simulink model "FormulaElectric"  (R2015a)
settings: Solver=ode1  StartTime=0.0  StopTime=inf  FixedStep=0.001  RelTol=1e-3
InitFcn:
  | %init_dyn_platform
  | FEParameters
StartFcn:
  | tic
StopFcn:
  | toc
undefined symbols (not defined in the file): Battery, Env, magnitude, Motor, RPM2Rad
libraries: vehicleLib x22, mblibv1 x15, driveline x12, fl_lib x8, simulink x6, AMKMotor x4, nesl_utility x4, WheelAssembly x4, ephysenetlib x2, ControllerLib x1, simulink_extras x1
(part 3 of 4)

== system FormulaElectric/Vehicle_model/Import Parameters ==
  Bus Creator1 : BusCreator  Inputs=934
  S-Function : S-Function  FunctionName=carparameters
      mask Display:
      | A=fileread('carparameters.h');
      | p=0;
      | namen=[];
      | for k=4:length(A)-5;
      |     if strcmp(A(k:k+4),'float')&~strcmp(A(k-3:k+4),'// float')&~strcmp(A(k-2:k+4),'//float')
      |         l=0;
      |         isfound=0;
      |         while ~isfound
      |             l=l+1;
      |             isfound=strcmp(A(k+l),';');
      |         end %while
      |         name=A(k+6:k+l-1);
      |         if strcmp(A(k+l-20:k+l-1),'[CAR_PARAM_MAXWHEEL]');
      |             name=A(k+6:k+l-21);
      |             for m=0:3
      |                 p=p+1;
      |                 port_label('output',p,[name,num2str(m)])
      |             end %for
      |         elseif strcmp(A(k+l-3:k+l-1),'[3]');
      |             name=A(k+6:k+l-4);
      |             p=p+1;
      |                 port_label('output',p,[name,'x'])
      |             p=p+1;
      |                 port_label('output',p,[name,'y'])
      |             p=p+1;
      |                 port_label('output',p,[name,'z'])
      |         elseif strcmp(A(k+l-3:k+l-1),'[7]');
      |             name=A(k+6:k+l-4);
      |             for m=0:6
      |                 p=p+1;
      |                 port_label('output',p,[name,num2str(m)])
      |             end
      |         elseif strcmp(A(k+l-16:k+l-1),'[INERTIA_TENSOR]');
      |             if  strcmp(A(k+l-36:k+l-1),'[CAR_PARAM_MAXWHEEL][INERTIA_TENSOR]');
      |             name=A(k+6:k+l-37);
      |             for n=0:3
      |             for m=0:5
      |                 p=p+1;
      |                 port_label('output',p,[name,num2str(n),num2str(m)])
      |             end
      |             end
      |             else
      |             name=A(k+6:k+l-17);
      |             for m=0:5
      |                 p=p+1;
      |                 port_label('output',p,[name,num2str(m)])
      |             end
      |             end %if
      |         elseif strcmp(A(k+l-20:k+l-1),'[PLANKPOINTS][THREE]');
      |             name=A(k+6:k+l-21);
      |             for m=0:7
      |             p=p+1;
      |                 port_label('output',p,[name,num2str(m),'x'])
      |             p=p+1;
      |                 port_label('output',p,[name,num2str(m),'y'])
      |             p=p+1;
      |                 port_label('output',p,[name,num2str(m),'z'])
      |             end
      |         else
      |         p=p+1;
      |         port_label('output',p,name)
      |         end %if
      |         %port_label('output',p,name)
      |     end %if
      | end %for
  imPar : Outport
  wires:
  S-Function/8 -> Bus Creator1/8  "aeroRefArea"
  S-Function/934 -> Bus Creator1/934  "test5"
  S-Function/933 -> Bus Creator1/933  "test4"
  S-Function/932 -> Bus Creator1/932  "test3"
  S-Function/931 -> Bus Creator1/931  "test2"
  S-Function/927 -> Bus Creator1/927  "suspThresholdDeg1"
  S-Function/928 -> Bus Creator1/928  "suspThresholdDeg2"
  S-Function/929 -> Bus Creator1/929  "suspThresholdDeg3"
  S-Function/930 -> Bus Creator1/930  "test1"
  S-Function/1 -> Bus Creator1/1  "bodyMass"
  S-Function/2 -> Bus Creator1/2  "bodyIxx"
  S-Function/3 -> Bus Creator1/3  "bodyIyy"
  S-Function/4 -> Bus Creator1/4  "bodyIzz"
  S-Function/5 -> Bus Creator1/5  "totVehMass"
  S-Function/6 -> Bus Creator1/6  "bodyCGz"
  S-Function/7 -> Bus Creator1/7  "aeroRho"
  S-Function/9 -> Bus Creator1/9  "aeroRefCX"
  S-Function/10 -> Bus Creator1/10  "aeroRefCZF"
  S-Function/11 -> Bus Creator1/11  "aeroRefCZR"
  S-Function/12 -> Bus Creator1/12  "aeroRefRHF"
  S-Function/13 -> Bus Creator1/13  "aeroRefRHR"
  S-Function/14 -> Bus Creator1/14  "aeroPxF"
  S-Function/15 -> Bus Creator1/15  "aeroPyF"
  S-Function/16 -> Bus Creator1/16  "aeroPzF"
  S-Function/18 -> Bus Creator1/18  "aeroPyR"
  S-Function/19 -> Bus Creator1/19  "aeroPzR"
  S-Function/20 -> Bus Creator1/20  "brakeBiasRatio"
  S-Function/21 -> Bus Creator1/21  "brakeMaxP"
  S-Function/22 -> Bus Creator1/22  "brakeDMasterF"
  S-Function/23 -> Bus Creator1/23  "brakeDiF"
  S-Function/24 -> Bus Creator1/24  "brakeDoF"
  S-Function/25 -> Bus Creator1/25  "brakeMuF"
  S-Function/26 -> Bus Creator1/26  "brakeBiasRatioF"
  S-Function/27 -> Bus Creator1/27  "brakeTCapF"
  S-Function/28 -> Bus Creator1/28  "brakeT0F"
  S-Function/29 -> Bus Creator1/29  "brakeTConF"
  S-Function/30 -> Bus Creator1/30  "brakeDCalF"
  S-Function/31 -> Bus Creator1/31  "brakeDiR"
  S-Function/32 -> Bus Creator1/32  "brakeDoR"
  S-Function/33 -> Bus Creator1/33  "brakeMuR"
  S-Function/34 -> Bus Creator1/34  "brakeBiasRatioR"
  S-Function/35 -> Bus Creator1/35  "brakeTCapR"
  S-Function/36 -> Bus Creator1/36  "brakeT0R"
  S-Function/37 -> Bus Creator1/37  "brakeTConR"
  S-Function/38 -> Bus Creator1/38  "brakeDCalR"
  S-Function/39 -> Bus Creator1/39  "steerR"
  S-Function/40 -> Bus Creator1/40  "steerPinionR"
  S-Function/41 -> Bus Creator1/41  "steerLeftMax"
  S-Function/42 -> Bus Creator1/42  "steerRightMax"
  S-Function/43 -> Bus Creator1/43  "steerDamper"
  S-Function/44 -> Bus Creator1/44  "steerStiff"
  S-Function/45 -> Bus Creator1/45  "steerPowerA"
  S-Function/46 -> Bus Creator1/46  "steerPowerTc"
  S-Function/47 -> Bus Creator1/47  "steerPMin"
  S-Function/48 -> Bus Creator1/48  "steerPMax"
  S-Function/49 -> Bus Creator1/49  "steerPowerZoneLeft"
  S-Function/50 -> Bus Creator1/50  "steerPowerZoneRight"
  S-Function/51 -> Bus Creator1/51  "engineMass"
  S-Function/52 -> Bus Creator1/52  "engineInertiaXX"
  S-Function/53 -> Bus Creator1/53  "engineInertiaYY"
  S-Function/54 -> Bus Creator1/54  "engineInertiaZZ"
  S-Function/55 -> Bus Creator1/55  "engineDamp"
  S-Function/56 -> Bus Creator1/56  "engineIdleSp"
  S-Function/57 -> Bus Creator1/57  "engineMaxTorq"
  S-Function/58 -> Bus Creator1/58  "clutchFCloseUp"
  S-Function/59 -> Bus Creator1/59  "clutchFCloseDown"
  S-Function/60 -> Bus Creator1/60  "clutchNbPlates"
  S-Function/61 -> Bus Creator1/61  "gearNbGears"
  S-Function/62 -> Bus Creator1/62  "gearEff"
  S-Function/63 -> Bus Creator1/63  "gearShiftTimeUp"
  S-Function/64 -> Bus Creator1/64  "gearShiftTimeDown"
  S-Function/65 -> Bus Creator1/65  "gearRatioPrim"
  S-Function/66 -> Bus Creator1/66  "gearRatio0"
  S-Function/67 -> Bus Creator1/67  "gearRatio1"
  S-Function/68 -> Bus Creator1/68  "gearRatio2"
  S-Function/69 -> Bus Creator1/69  "gearRatio3"
  S-Function/70 -> Bus Creator1/70  "gearRatio4"
  S-Function/71 -> Bus Creator1/71  "gearRatio5"
  S-Function/72 -> Bus Creator1/72  "gearRatio6"
  S-Function/73 -> Bus Creator1/73  "gearRatio7"
  S-Function/74 -> Bus Creator1/74  "diffType0"
  S-Function/75 -> Bus Creator1/75  "diffType1"
  S-Function/76 -> Bus Creator1/76  "diffType2"
  S-Function/77 -> Bus Creator1/77  "diffRatio0"
  S-Function/78 -> Bus Creator1/78  "diffRatio1"
  S-Function/79 -> Bus Creator1/79  "diffRatio2"
  S-Function/80 -> Bus Creator1/80  "diffPAngle0"
  S-Function/81 -> Bus Creator1/81  "diffPAngle1"
  S-Function/82 -> Bus Creator1/82  "diffPAngle2"
  S-Function/83 -> Bus Creator1/83  "diffCAngle0"
  S-Function/84 -> Bus Creator1/84  "diffCAngle1"
  S-Function/85 -> Bus Creator1/85  "diffCAngle2"
  S-Function/86 -> Bus Creator1/86  "diffClutch0"
  S-Function/87 -> Bus Creator1/87  "diffClutch1"
  S-Function/88 -> Bus Creator1/88  "diffClutch2"
  S-Function/89 -> Bus Creator1/89  "diffLock0"
  S-Function/90 -> Bus Creator1/90  "diffLock1"
  S-Function/91 -> Bus Creator1/91  "diffLock2"
  S-Function/92 -> Bus Creator1/92  "suspStiff0"
  S-Function/93 -> Bus Creator1/93  "suspStiff1"
  S-Function/94 -> Bus Creator1/94  "suspStiff2"
  S-Function/95 -> Bus Creator1/95  "suspStiff3"
  S-Function/96 -> Bus Creator1/96  "suspSpringRestLength0"
  S-Function/97 -> Bus Creator1/97  "suspSpringRestLength1"
  S-Function/98 -> Bus Creator1/98  "suspSpringRestLength2"
  S-Function/99 -> Bus Creator1/99  "suspSpringRestLength3"
  S-Function/100 -> Bus Creator1/100  "suspDamp0"
  S-Function/101 -> Bus Creator1/101  "suspDamp1"
  S-Function/102 -> Bus Creator1/102  "suspDamp2"
  S-Function/103 -> Bus Creator1/103  "suspDamp3"
  S-Function/104 -> Bus Creator1/104  "suspDampLength0"
  S-Function/105 -> Bus Creator1/105  "suspDampLength1"
  S-Function/106 -> Bus Creator1/106  "suspDampLength2"
  S-Function/107 -> Bus Creator1/107  "suspDampLength3"
  S-Function/108 -> Bus Creator1/108  "suspRimMass0"
  S-Function/109 -> Bus Creator1/109  "suspRimMass1"
  S-Function/110 -> Bus Creator1/110  "suspRimMass2"
  S-Function/111 -> Bus Creator1/111  "suspRimMass3"
  S-Function/112 -> Bus Creator1/112  "suspRimRadius0"
  S-Function/113 -> Bus Creator1/113  "suspRimRadius1"
  S-Function/114 -> Bus Creator1/114  "suspRimRadius2"
  S-Function/115 -> Bus Creator1/115  "suspRimRadius3"
  S-Function/116 -> Bus Creator1/116  "suspRimInertiaXX0"
  S-Function/117 -> Bus Creator1/117  "suspRimInertiaXX1"
  S-Function/118 -> Bus Creator1/118  "suspRimInertiaXX2"
  S-Function/119 -> Bus Creator1/119  "suspRimInertiaXX3"
  S-Function/120 -> Bus Creator1/120  "suspRimInertiaYY0"
  S-Function/121 -> Bus Creator1/121  "suspRimInertiaYY1"
  S-Function/122 -> Bus Creator1/122  "suspRimInertiaYY2"
  S-Function/123 -> Bus Creator1/123  "suspRimInertiaYY3"
  S-Function/124 -> Bus Creator1/124  "suspRimInertiaZZ0"
  S-Function/125 -> Bus Creator1/125  "suspRimInertiaZZ1"
  S-Function/126 -> Bus Creator1/126  "suspRimInertiaZZ2"
  S-Function/127 -> Bus Creator1/127  "suspRimInertiaZZ3"
  S-Function/128 -> Bus Creator1/128  "suspCamber0"
  S-Function/129 -> Bus Creator1/129  "suspCamber1"
  S-Function/130 -> Bus Creator1/130  "suspCamber2"
  S-Function/131 -> Bus Creator1/131  "suspCamber3"
  S-Function/132 -> Bus Creator1/132  "suspCaster0"
  S-Function/133 -> Bus Creator1/133  "suspCaster1"
  S-Function/134 -> Bus Creator1/134  "suspCaster2"
  S-Function/135 -> Bus Creator1/135  "suspCaster3"
  S-Function/136 -> Bus Creator1/136  "suspToe0"
  S-Function/137 -> Bus Creator1/137  "suspToe1"
  S-Function/138 -> Bus Creator1/138  "suspToe2"
  S-Function/139 -> Bus Creator1/139  "suspToe3"
  S-Function/140 -> Bus Creator1/140  "suspRH0"
  S-Function/141 -> Bus Creator1/141  "suspRH1"
  S-Function/142 -> Bus Creator1/142  "suspRH2"
  S-Function/143 -> Bus Creator1/143  "suspRH3"
  S-Function/144 -> Bus Creator1/144  "suspTr0"
  S-Function/145 -> Bus Creator1/145  "suspTr1"
  S-Function/146 -> Bus Creator1/146  "suspTr2"
  S-Function/147 -> Bus Creator1/147  "suspTr3"
  S-Function/148 -> Bus Creator1/148  "suspPrel0"
  S-Function/149 -> Bus Creator1/149  "suspPrel1"
  S-Function/150 -> Bus Creator1/150  "suspPrel2"
  S-Function/151 -> Bus Creator1/151  "suspPrel3"
  S-Function/152 -> Bus Creator1/152  "suspAttFz"
  S-Function/153 -> Bus Creator1/153  "suspAttRz"
  S-Function/154 -> Bus Creator1/154  "suspRollCF"
  S-Function/155 -> Bus Creator1/155  "suspRollCR"
  S-Function/156 -> Bus Creator1/156  "suspRollPosF"
  S-Function/157 -> Bus Creator1/157  "suspRollPosR"
  S-Function/158 -> Bus Creator1/158  "tyreMass0"
  S-Function/159 -> Bus Creator1/159  "tyreMass1"
  S-Function/160 -> Bus Creator1/160  "tyreMass2"
  S-Function/161 -> Bus Creator1/161  "tyreMass3"
  S-Function/162 -> Bus Creator1/162  "tyreRadius0"
  S-Function/163 -> Bus Creator1/163  "tyreRadius1"
  S-Function/164 -> Bus Creator1/164  "tyreRadius2"
  S-Function/165 -> Bus Creator1/165  "tyreRadius3"
  S-Function/166 -> Bus Creator1/166  "tyreInertiaXX0"
  S-Function/167 -> Bus Creator1/167  "tyreInertiaXX1"
  S-Function/168 -> Bus Creator1/168  "tyreInertiaXX2"
  S-Function/169 -> Bus Creator1/169  "tyreInertiaXX3"
  S-Function/170 -> Bus Creator1/170  "tyreInertiaYY0"
  S-Function/171 -> Bus Creator1/171  "tyreInertiaYY1"
  S-Function/172 -> Bus Creator1/172  "tyreInertiaYY2"
  S-Function/173 -> Bus Creator1/173  "tyreInertiaYY3"
  S-Function/174 -> Bus Creator1/174  "tyreInertiaZZ0"
  S-Function/175 -> Bus Creator1/175  "tyreInertiaZZ1"
  S-Function/176 -> Bus Creator1/176  "tyreInertiaZZ2"
  S-Function/177 -> Bus Creator1/177  "tyreInertiaZZ3"
  S-Function/178 -> Bus Creator1/178  "tyreLfz0f"
  S-Function/179 -> Bus Creator1/179  "tyreLcxf"
  S-Function/180 -> Bus Creator1/180  "tyreLmuxf"
  S-Function/181 -> Bus Creator1/181  "tyreLexf"
  S-Function/182 -> Bus Creator1/182  "tyreLkxf"
  S-Function/183 -> Bus Creator1/183  "tyreLhxf"
  S-Function/184 -> Bus Creator1/184  "tyreLvxf"
  S-Function/185 -> Bus Creator1/185  "tyreLcyf"
  S-Function/186 -> Bus Creator1/186  "tyreLmuyf"
  S-Function/187 -> Bus Creator1/187  "tyreLeyf"
  S-Function/188 -> Bus Creator1/188  "tyreLkyf"
  S-Function/189 -> Bus Creator1/189  "tyreLkycf"
  S-Function/190 -> Bus Creator1/190  "tyreLkzcf"
  S-Function/191 -> Bus Creator1/191  "tyreLhyf"
  S-Function/192 -> Bus Creator1/192  "tyreLvyf"
  S-Function/193 -> Bus Creator1/193  "tyreLtrf"
  S-Function/194 -> Bus Creator1/194  "tyreLresf"
  S-Function/195 -> Bus Creator1/195  "tyreLxalf"
  S-Function/196 -> Bus Creator1/196  "tyreLykaf"
  S-Function/197 -> Bus Creator1/197  "tyreLvykaf"
  S-Function/198 -> Bus Creator1/198  "tyreLsf"
  S-Function/199 -> Bus Creator1/199  "tyreLmxf"
  S-Function/200 -> Bus Creator1/200  "tyreLvmxf"
  S-Function/201 -> Bus Creator1/201  "tyreLmyf"
  S-Function/202 -> Bus Creator1/202  "tyreLmpf"
  S-Function/203 -> Bus Creator1/203  "tyreLsgkpf"
  S-Function/204 -> Bus Creator1/204  "tyreLsgalf"
  S-Function/205 -> Bus Creator1/205  "tyreLdampf"
  S-Function/206 -> Bus Creator1/206  "tyreLmassf"
  S-Function/207 -> Bus Creator1/207  "tyreLInertiaf"
  S-Function/208 -> Bus Creator1/208  "tyreEnableChkF"
  S-Function/209 -> Bus Creator1/209  "tyreEnableSatF"
  S-Function/210 -> Bus Creator1/210  "tyreEnableTempF"
  S-Function/211 -> Bus Creator1/211  "tyreTempAF"
  S-Function/212 -> Bus Creator1/212  "tyreTempBF"
  S-Function/213 -> Bus Creator1/213  "tyreLfz0r"
  S-Function/214 -> Bus Creator1/214  "tyreLcxr"
  S-Function/215 -> Bus Creator1/215  "tyreLmuxr"
  S-Function/216 -> Bus Creator1/216  "tyreLexr"
  S-Function/217 -> Bus Creator1/217  "tyreLkxr"
  S-Function/218 -> Bus Creator1/218  "tyreLhxr"
  S-Function/219 -> Bus Creator1/219  "tyreLvxr"
  S-Function/220 -> Bus Creator1/220  "tyreLcyr"
  S-Function/221 -> Bus Creator1/221  "tyreLmuyr"
  S-Function/222 -> Bus Creator1/222  "tyreLeyr"
  S-Function/223 -> Bus Creator1/223  "tyreLkyr"
  S-Function/224 -> Bus Creator1/224  "tyreLkycr"
  S-Function/225 -> Bus Creator1/225  "tyreLkzcr"
  S-Function/226 -> Bus Creator1/226  "tyreLhyr"
  S-Function/227 -> Bus Creator1/227  "tyreLvyr"
  S-Function/228 -> Bus Creator1/228  "tyreLtrr"
  S-Function/229 -> Bus Creator1/229  "tyreLresr"
  S-Function/230 -> Bus Creator1/230  "tyreLxalr"
  S-Function/231 -> Bus Creator1/231  "tyreLykar"
  S-Function/232 -> Bus Creator1/232  "tyreLvykar"
  S-Function/233 -> Bus Creator1/233  "tyreLsr"
  S-Function/234 -> Bus Creator1/234  "tyreLmxr"
  S-Function/235 -> Bus Creator1/235  "tyreLvmxr"
  S-Function/236 -> Bus Creator1/236  "tyreLmyr"
  S-Function/237 -> Bus Creator1/237  "tyreLmpr"
  S-Function/238 -> Bus Creator1/238  "tyreLsgkpr"
  S-Function/239 -> Bus Creator1/239  "tyreLsgalr"
  S-Function/240 -> Bus Creator1/240  "tyreLdampr"
  S-Function/241 -> Bus Creator1/241  "tyreLmassr"
  S-Function/242 -> Bus Creator1/242  "tyreLInertiar"
  S-Function/243 -> Bus Creator1/243  "tyreEnableChkR"
  S-Function/244 -> Bus Creator1/244  "tyreEnableSatR"
  S-Function/245 -> Bus Creator1/245  "tyreEnableTempR"
  S-Function/246 -> Bus Creator1/246  "tyreTempAR"
  S-Function/247 -> Bus Creator1/247  "tyreTempBR"
  S-Function/248 -> Bus Creator1/248  "CSantiStallMode"
  S-Function/249 -> Bus Creator1/249  "CSantiStallEnable"
  S-Function/250 -> Bus Creator1/250  "CSantiStallRPM"
  S-Function/251 -> Bus Creator1/251  "CSantiStallTime"
  S-Function/252 -> Bus Creator1/252  "CStracContrKp"
  S-Function/253 -> Bus Creator1/253  "CStracContrKi"
  S-Function/254 -> Bus Creator1/254  "CStracContrMinVel"
  S-Function/255 -> Bus Creator1/255  "CSthrPulseEnableUp"
  S-Function/256 -> Bus Creator1/256  "CSthrPulseEnableDown"
  S-Function/257 -> Bus Creator1/257  "CSthrPulseKp"
  S-Function/258 -> Bus Creator1/258  "CSthrPulseKi"
  S-Function/259 -> Bus Creator1/259  "CSidleConThrLim"
  S-Function/260 -> Bus Creator1/260  "CSidleConRPM"
  S-Function/261 -> Bus Creator1/261  "CSidleConMinRPM"
  S-Function/262 -> Bus Creator1/262  "CSidleConMaxRPM"
  S-Function/263 -> Bus Creator1/263  "CSidleConKp"
  S-Function/264 -> Bus Creator1/264  "CSidleConKi"
  S-Function/17 -> Bus Creator1/17  "aeroPxR"
  S-Function/265 -> Bus Creator1/265  "CSpitLimVel"
  S-Function/266 -> Bus Creator1/266  "skidLongF"
  S-Function/267 -> Bus Creator1/267  "skidLatF"
  S-Function/268 -> Bus Creator1/268  "skidLongR"
  S-Function/269 -> Bus Creator1/269  "skidLatR"
  S-Function/270 -> Bus Creator1/270  "clutchMaxPedalDispl"
  S-Function/271 -> Bus Creator1/271  "clutchMaxDispl"
  S-Function/272 -> Bus Creator1/272  "clutchFOpenUp"
  S-Function/273 -> Bus Creator1/273  "clutchFOpenDown"
  S-Function/274 -> Bus Creator1/274  "clutchEnableUp"
  S-Function/275 -> Bus Creator1/275  "clutchEnableDown"
  S-Function/276 -> Bus Creator1/276  "gearFactor"
  S-Function/277 -> Bus Creator1/277  "gearEnableAuto"
  S-Function/278 -> Bus Creator1/278  "gearEnableRev"
  S-Function/279 -> Bus Creator1/279  "diffEnable0"
  S-Function/281 -> Bus Creator1/281  "diffEnable2"
  S-Function/280 -> Bus Creator1/280  "diffEnable1"
  S-Function/282 -> Bus Creator1/282  "diffPreload0"
  S-Function/283 -> Bus Creator1/283  "diffPreload1"
  S-Function/284 -> Bus Creator1/284  "diffPreload2"
  S-Function/285 -> Bus Creator1/285  "satRadius0"
  S-Function/286 -> Bus Creator1/286  "satRadius1"
  S-Function/287 -> Bus Creator1/287  "satRadius2"
  S-Function/288 -> Bus Creator1/288  "maxTorq0"
  S-Function/289 -> Bus Creator1/289  "maxTorq1"
  S-Function/290 -> Bus Creator1/290  "maxTorq2"
  S-Function/291 -> Bus Creator1/291  "tyrePressF"
  S-Function/292 -> Bus Creator1/292  "tyrePressR"
  S-Function/293 -> Bus Creator1/293  "steerEnableLock"
  S-Function/294 -> Bus Creator1/294  "steerAngleLock"
  S-Function/295 -> Bus Creator1/295  "steerOffset"
  S-Function/296 -> Bus Creator1/296  "suspDampBumpSet0"
  S-Function/297 -> Bus Creator1/297  "suspDampBumpSet1"
  S-Function/298 -> Bus Creator1/298  "suspDampBumpSet2"
  S-Function/299 -> Bus Creator1/299  "suspDampBumpSet3"
  S-Function/300 -> Bus Creator1/300  "suspDampReboundSet0"
  S-Function/301 -> Bus Creator1/301  "suspDampReboundSet1"
  S-Function/302 -> Bus Creator1/302  "suspDampReboundSet2"
  S-Function/303 -> Bus Creator1/303  "suspDampReboundSet3"
  S-Function/304 -> Bus Creator1/304  "suspCentralBumpStopGapF"
  S-Function/305 -> Bus Creator1/305  "suspBumpStopGapF"
  S-Function/306 -> Bus Creator1/306  "suspCentralBumpStopGapR"
  S-Function/307 -> Bus Creator1/307  "suspBumpStopGapR"
  S-Function/308 -> Bus Creator1/308  "suspEnableBumpStopF"
  S-Function/309 -> Bus Creator1/309  "suspEnableBumpStopR"
  S-Function/310 -> Bus Creator1/310  "suspEnableCentralBumpStopF"
  S-Function/311 -> Bus Creator1/311  "suspEnableCentralBumpStopR"
  S-Function/312 -> Bus Creator1/312  "suspBumpStopF0"
  S-Function/313 -> Bus Creator1/313  "suspBumpStopF1"
  S-Function/314 -> Bus Creator1/314  "suspBumpStopF2"
  S-Function/315 -> Bus Creator1/315  "suspBumpStopF3"
  S-Function/316 -> Bus Creator1/316  "suspBumpStopF4"
  S-Function/317 -> Bus Creator1/317  "suspBumpStopF5"
  S-Function/318 -> Bus Creator1/318  "suspBumpStopF6"
  S-Function/319 -> Bus Creator1/319  "suspBumpStopR0"
  S-Function/320 -> Bus Creator1/320  "suspBumpStopR1"
  S-Function/321 -> Bus Creator1/321  "suspBumpStopR2"
  S-Function/322 -> Bus Creator1/322  "suspBumpStopR3"
  S-Function/323 -> Bus Creator1/323  "suspBumpStopR4"
  S-Function/324 -> Bus Creator1/324  "suspBumpStopR5"
  S-Function/325 -> Bus Creator1/325  "suspBumpStopR6"
  S-Function/326 -> Bus Creator1/326  "gearDelayDown"
  S-Function/327 -> Bus Creator1/327  "gearDelayUp"
  S-Function/328 -> Bus Creator1/328  "tyreTCapF"
  S-Function/329 -> Bus Creator1/329  "tyreTambF"
  S-Function/330 -> Bus Creator1/330  "tyreTConAmbF"
  S-Function/331 -> Bus Creator1/331  "tyreTCapR"
  S-Function/332 -> Bus Creator1/332  "tyreTambR"
  S-Function/333 -> Bus Creator1/333  "tyreTConAmbR"
  S-Function/334 -> Bus Creator1/334  "brakeDMasterR"
  S-Function/335 -> Bus Creator1/335  "scaleAccX"
  S-Function/336 -> Bus Creator1/336  "scaleAccY"
  S-Function/337 -> Bus Creator1/337  "scaleAccZ"
  S-Function/338 -> Bus Creator1/338  "suspDampPrel0"
  S-Function/339 -> Bus Creator1/339  "suspDampPrel1"
  S-Function/343 -> Bus Creator1/343  "brakeCalGainF"
  S-Function/342 -> Bus Creator1/342  "brakeCalOffsetF"
  S-Function/341 -> Bus Creator1/341  "suspDampPrel3"
  S-Function/340 -> Bus Creator1/340  "suspDampPrel2"
  S-Function/344 -> Bus Creator1/344  "brakeCalOffsetR"
  S-Function/345 -> Bus Creator1/345  "brakeCalGainR"
  S-Function/346 -> Bus Creator1/346  "bodyCGx"
  S-Function/347 -> Bus Creator1/347  "bodyCGy"
  S-Function/348 -> Bus Creator1/348  "suspBumpCenStopF0"
  S-Function/349 -> Bus Creator1/349  "suspBumpCenStopF1"
  S-Function/365 -> Bus Creator1/365  "warpLen1"
  S-Function/364 -> Bus Creator1/364  "warpLen0"
  S-Function/363 -> Bus Creator1/363  "suspAttRx"
  S-Function/362 -> Bus Creator1/362  "suspAttFx"
  S-Function/361 -> Bus Creator1/361  "suspBumpCenStopR6"
  S-Function/360 -> Bus Creator1/360  "suspBumpCenStopR5"
  S-Function/359 -> Bus Creator1/359  "suspBumpCenStopR4"
  S-Function/358 -> Bus Creator1/358  "suspBumpCenStopR3"
  S-Function/357 -> Bus Creator1/357  "suspBumpCenStopR2"
  S-Function/356 -> Bus Creator1/356  "suspBumpCenStopR1"
  S-Function/355 -> Bus Creator1/355  "suspBumpCenStopR0"
  S-Function/354 -> Bus Creator1/354  "suspBumpCenStopF6"
  S-Function/353 -> Bus Creator1/353  "suspBumpCenStopF5"
  S-Function/352 -> Bus Creator1/352  "suspBumpCenStopF4"
  S-Function/351 -> Bus Creator1/351  "suspBumpCenStopF3"
  S-Function/350 -> Bus Creator1/350  "suspBumpCenStopF2"
  S-Function/366 -> Bus Creator1/366  "warpLen2"
  S-Function/367 -> Bus Creator1/367  "warpLen3"
  S-Function/368 -> Bus Creator1/368  "tyreWidth0"
  S-Function/369 -> Bus Creator1/369  "tyreWidth1"
  S-Function/370 -> Bus Creator1/370  "tyreWidth2"
  S-Function/371 -> Bus Creator1/371  "tyreWidth3"
  S-Function/372 -> Bus Creator1/372  "suspPoint1Fx"
  S-Function/373 -> Bus Creator1/373  "suspPoint1Fy"
  S-Function/374 -> Bus Creator1/374  "suspPoint1Fz"
  S-Function/376 -> Bus Creator1/376  "suspPoint2Fy"
  S-Function/375 -> Bus Creator1/375  "suspPoint2Fx"
  S-Function/377 -> Bus Creator1/377  "suspPoint2Fz"
  S-Function/378 -> Bus Creator1/378  "suspPoint3Fx"
  S-Function/379 -> Bus Creator1/379  "suspPoint3Fy"
  S-Function/380 -> Bus Creator1/380  "suspPoint3Fz"
  S-Function/381 -> Bus Creator1/381  "suspPoint4Fx"
  S-Function/382 -> Bus Creator1/382  "suspPoint4Fy"
  S-Function/383 -> Bus Creator1/383  "suspPoint4Fz"
  S-Function/384 -> Bus Creator1/384  "suspPoint5Fx"
  S-Function/385 -> Bus Creator1/385  "suspPoint5Fy"
  S-Function/386 -> Bus Creator1/386  "suspPoint5Fz"
  S-Function/387 -> Bus Creator1/387  "suspPoint6Fx"
  S-Function/389 -> Bus Creator1/389  "suspPoint6Fz"
  S-Function/388 -> Bus Creator1/388  "suspPoint6Fy"
  S-Function/390 -> Bus Creator1/390  "suspPoint7Fx"
  S-Function/391 -> Bus Creator1/391  "suspPoint7Fy"
  S-Function/393 -> Bus Creator1/393  "suspPoint8Fx"
  S-Function/394 -> Bus Creator1/394  "suspPoint8Fy"
  S-Function/395 -> Bus Creator1/395  "suspPoint8Fz"
  S-Function/396 -> Bus Creator1/396  "suspPoint9Fx"
  S-Function/397 -> Bus Creator1/397  "suspPoint9Fy"
  S-Function/398 -> Bus Creator1/398  "suspPoint9Fz"
  S-Function/399 -> Bus Creator1/399  "suspPoint10Fx"
  S-Function/400 -> Bus Creator1/400  "suspPoint10Fy"
  S-Function/401 -> Bus Creator1/401  "suspPoint10Fz"
  S-Function/402 -> Bus Creator1/402  "suspPoint11Fx"
  S-Function/403 -> Bus Creator1/403  "suspPoint11Fy"
  S-Function/404 -> Bus Creator1/404  "suspPoint11Fz"
  S-Function/405 -> Bus Creator1/405  "suspPoint12Fx"
  S-Function/406 -> Bus Creator1/406  "suspPoint12Fy"
  S-Function/407 -> Bus Creator1/407  "suspPoint12Fz"
  S-Function/408 -> Bus Creator1/408  "suspPoint13bottomFx"
  S-Function/409 -> Bus Creator1/409  "suspPoint13bottomFy"
  S-Function/410 -> Bus Creator1/410  "suspPoint13bottomFz"
  S-Function/411 -> Bus Creator1/411  "suspPoint13topFx"
  S-Function/412 -> Bus Creator1/412  "suspPoint13topFy"
  S-Function/413 -> Bus Creator1/413  "suspPoint13topFz"
  S-Function/414 -> Bus Creator1/414  "suspPoint14Fx"
  S-Function/415 -> Bus Creator1/415  "suspPoint14Fy"
  S-Function/416 -> Bus Creator1/416  "suspPoint14Fz"
  S-Function/417 -> Bus Creator1/417  "suspPoint15Fx"
  S-Function/418 -> Bus Creator1/418  "suspPoint15Fy"
  S-Function/419 -> Bus Creator1/419  "suspPoint15Fz"
  S-Function/420 -> Bus Creator1/420  "suspPoint17Fx"
  S-Function/421 -> Bus Creator1/421  "suspPoint17Fy"
  S-Function/422 -> Bus Creator1/422  "suspPoint17Fz"
  S-Function/423 -> Bus Creator1/423  "suspPoint19Fx"
  S-Function/424 -> Bus Creator1/424  "suspPoint19Fy"
  S-Function/425 -> Bus Creator1/425  "suspPoint19Fz"
  S-Function/426 -> Bus Creator1/426  "suspPoint20Fx"
  S-Function/427 -> Bus Creator1/427  "suspPoint20Fy"
  S-Function/428 -> Bus Creator1/428  "suspPoint20Fz"
  S-Function/429 -> Bus Creator1/429  "suspPoint21Fx"
  S-Function/430 -> Bus Creator1/430  "suspPoint21Fy"
  S-Function/431 -> Bus Creator1/431  "suspPoint21Fz"
  S-Function/432 -> Bus Creator1/432  "suspPoint30Fx"
  S-Function/433 -> Bus Creator1/433  "suspPoint30Fy"
  S-Function/434 -> Bus Creator1/434  "suspPoint30Fz"
  S-Function/435 -> Bus Creator1/435  "suspPoint31Fx"
  S-Function/436 -> Bus Creator1/436  "suspPoint31Fy"
  S-Function/437 -> Bus Creator1/437  "suspPoint31Fz"
  S-Function/438 -> Bus Creator1/438  "suspPoint1Rx"
  S-Function/439 -> Bus Creator1/439  "suspPoint1Ry"
  S-Function/440 -> Bus Creator1/440  "suspPoint1Rz"
  S-Function/441 -> Bus Creator1/441  "suspPoint2Rx"
  S-Function/442 -> Bus Creator1/442  "suspPoint2Ry"
  S-Function/443 -> Bus Creator1/443  "suspPoint2Rz"
  S-Function/444 -> Bus Creator1/444  "suspPoint3Rx"
  S-Function/445 -> Bus Creator1/445  "suspPoint3Ry"
  S-Function/446 -> Bus Creator1/446  "suspPoint3Rz"
  S-Function/447 -> Bus Creator1/447  "suspPoint4Rx"
  S-Function/448 -> Bus Creator1/448  "suspPoint4Ry"
  S-Function/449 -> Bus Creator1/449  "suspPoint4Rz"
  S-Function/450 -> Bus Creator1/450  "suspPoint5Rx"
  S-Function/451 -> Bus Creator1/451  "suspPoint5Ry"
  S-Function/452 -> Bus Creator1/452  "suspPoint5Rz"
  S-Function/453 -> Bus Creator1/453  "suspPoint6Rx"
  S-Function/454 -> Bus Creator1/454  "suspPoint6Ry"
  S-Function/455 -> Bus Creator1/455  "suspPoint6Rz"
  S-Function/456 -> Bus Creator1/456  "suspPoint7Rx"
  S-Function/457 -> Bus Creator1/457  "suspPoint7Ry"
  S-Function/458 -> Bus Creator1/458  "suspPoint7Rz"
  S-Function/459 -> Bus Creator1/459  "suspPoint8Rx"
  S-Function/460 -> Bus Creator1/460  "suspPoint8Ry"
  S-Function/461 -> Bus Creator1/461  "suspPoint8Rz"
  S-Function/462 -> Bus Creator1/462  "suspPoint9Rx"
  S-Function/463 -> Bus Creator1/463  "suspPoint9Ry"
  S-Function/464 -> Bus Creator1/464  "suspPoint9Rz"
  S-Function/465 -> Bus Creator1/465  "suspPoint10Rx"
  S-Function/466 -> Bus Creator1/466  "suspPoint10Ry"
  S-Function/467 -> Bus Creator1/467  "suspPoint10Rz"
  S-Function/468 -> Bus Creator1/468  "suspPoint11Rx"
  S-Function/469 -> Bus Creator1/469  "suspPoint11Ry"
  S-Function/470 -> Bus Creator1/470  "suspPoint11Rz"
  S-Function/471 -> Bus Creator1/471  "suspPoint12Rx"
  S-Function/472 -> Bus Creator1/472  "suspPoint12Ry"
  S-Function/473 -> Bus Creator1/473  "suspPoint12Rz"
  S-Function/474 -> Bus Creator1/474  "suspPoint13bottomRx"
  S-Function/475 -> Bus Creator1/475  "suspPoint13bottomRy"
  S-Function/476 -> Bus Creator1/476  "suspPoint13bottomRz"
  S-Function/477 -> Bus Creator1/477  "suspPoint13topRx"
  S-Function/478 -> Bus Creator1/478  "suspPoint13topRy"
  S-Function/479 -> Bus Creator1/479  "suspPoint13topRz"
  S-Function/480 -> Bus Creator1/480  "suspPoint14Rx"
  S-Function/481 -> Bus Creator1/481  "suspPoint14Ry"
  S-Function/482 -> Bus Creator1/482  "suspPoint14Rz"
  S-Function/483 -> Bus Creator1/483  "suspPoint15Rx"
  S-Function/484 -> Bus Creator1/484  "suspPoint15Ry"
  S-Function/485 -> Bus Creator1/485  "suspPoint15Rz"
  S-Function/486 -> Bus Creator1/486  "suspPoint17Rx"
  S-Function/487 -> Bus Creator1/487  "suspPoint17Ry"
  S-Function/488 -> Bus Creator1/488  "suspPoint17Rz"
  S-Function/489 -> Bus Creator1/489  "suspPoint19Rx"
  S-Function/490 -> Bus Creator1/490  "suspPoint19Ry"
  S-Function/491 -> Bus Creator1/491  "suspPoint19Rz"
  S-Function/492 -> Bus Creator1/492  "suspPoint20Rx"
  S-Function/493 -> Bus Creator1/493  "suspPoint20Ry"
  S-Function/494 -> Bus Creator1/494  "suspPoint20Rz"
  S-Function/495 -> Bus Creator1/495  "suspPoint21Rx"
  S-Function/496 -> Bus Creator1/496  "suspPoint21Ry"
  S-Function/497 -> Bus Creator1/497  "suspPoint21Rz"
  S-Function/498 -> Bus Creator1/498  "suspPoint30Rx"
  S-Function/499 -> Bus Creator1/499  "suspPoint30Ry"
  S-Function/500 -> Bus Creator1/500  "suspPoint30Rz"
  S-Function/501 -> Bus Creator1/501  "suspPoint31Rx"
  S-Function/502 -> Bus Creator1/502  "suspPoint31Ry"
  S-Function/503 -> Bus Creator1/503  "suspPoint31Rz"
  S-Function/504 -> Bus Creator1/504  "suspRockerMass0"
  S-Function/505 -> Bus Creator1/505  "suspRockerMass1"
  S-Function/506 -> Bus Creator1/506  "suspRockerMass2"
  S-Function/507 -> Bus Creator1/507  "suspRockerMass3"
  S-Function/508 -> Bus Creator1/508  "suspUprightMass0"
  S-Function/509 -> Bus Creator1/509  "suspUprightMass1"
  S-Function/510 -> Bus Creator1/510  "suspUprightMass2"
  S-Function/511 -> Bus Creator1/511  "suspUprightMass3"
  S-Function/512 -> Bus Creator1/512  "steerrackMass"
  S-Function/513 -> Bus Creator1/513  "suspRollMassF"
  S-Function/514 -> Bus Creator1/514  "suspRollMassR"
  S-Function/515 -> Bus Creator1/515  "suspRollStepF"
  S-Function/516 -> Bus Creator1/516  "suspRollStepR"
  S-Function/392 -> Bus Creator1/392  "suspPoint7Fz"
  S-Function/517 -> Bus Creator1/517  "suspSnubberEnableF"
  S-Function/518 -> Bus Creator1/518  "suspSnubberEnableR"
  S-Function/519 -> Bus Creator1/519  "suspSnubberDampF"
  S-Function/520 -> Bus Creator1/520  "suspSnubberDampR"
  S-Function/521 -> Bus Creator1/521  "suspSnubberDeflMinF"
  S-Function/522 -> Bus Creator1/522  "suspSnubberDeflMinR"
  S-Function/523 -> Bus Creator1/523  "suspSnubberDeflMaxF"
  S-Function/524 -> Bus Creator1/524  "suspSnubberDeflMaxR"
  S-Function/525 -> Bus Creator1/525  "suspWeightBalance"
  S-Function/526 -> Bus Creator1/526  "enginePosx"
  S-Function/527 -> Bus Creator1/527  "enginePosy"
  S-Function/528 -> Bus Creator1/528  "enginePosz"
  S-Function/529 -> Bus Creator1/529  "fuelEnableMass"
  S-Function/530 -> Bus Creator1/530  "fuelEnableTank"
  S-Function/535 -> Bus Creator1/535  "fuelDensity"
  S-Function/534 -> Bus Creator1/534  "fuelCap"
  S-Function/533 -> Bus Creator1/533  "fuelRPMBSFC"
  S-Function/532 -> Bus Creator1/532  "fuelBSFC"
  S-Function/531 -> Bus Creator1/531  "fuelDesign"
  S-Function/536 -> Bus Creator1/536  "combModeF"
  S-Function/537 -> Bus Creator1/537  "combModeR"
  S-Function/538 -> Bus Creator1/538  "suspStaticCom0"
  S-Function/539 -> Bus Creator1/539  "suspStaticCom1"
  S-Function/540 -> Bus Creator1/540  "suspStaticCom2"
  S-Function/541 -> Bus Creator1/541  "suspStaticCom3"
  S-Function/542 -> Bus Creator1/542  "suspSprMinLen0"
  S-Function/543 -> Bus Creator1/543  "suspSprMinLen1"
  S-Function/544 -> Bus Creator1/544  "suspSprMinLen2"
  S-Function/545 -> Bus Creator1/545  "suspSprMinLen3"
  S-Function/546 -> Bus Creator1/546  "suspBearingFriction0"
  S-Function/547 -> Bus Creator1/547  "suspBearingFriction1"
  S-Function/548 -> Bus Creator1/548  "suspBearingFriction2"
  S-Function/549 -> Bus Creator1/549  "suspBearingFriction3"
  S-Function/550 -> Bus Creator1/550  "engineScaleRevLim"
  S-Function/551 -> Bus Creator1/551  "engineScalePitLim"
  S-Function/552 -> Bus Creator1/552  "engineScaleShift"
  S-Function/553 -> Bus Creator1/553  "aeroPxCOP"
  S-Function/554 -> Bus Creator1/554  "aeroPyCOP"
  S-Function/555 -> Bus Creator1/555  "aeroPzCOP"
  S-Function/556 -> Bus Creator1/556  "vWearF"
  S-Function/557 -> Bus Creator1/557  "nPowerWearF"
  S-Function/558 -> Bus Creator1/558  "nomTreadHeightF"
  S-Function/559 -> Bus Creator1/559  "alphaWFacF"
  S-Function/560 -> Bus Creator1/560  "kappaWFacF"
  S-Function/561 -> Bus Creator1/561  "camberWFacF"
  S-Function/562 -> Bus Creator1/562  "muxWEARF"
  S-Function/563 -> Bus Creator1/563  "ckappaWEARF"
  S-Function/564 -> Bus Creator1/564  "muyWEARF"
  S-Function/565 -> Bus Creator1/565  "cfalphaWEARF"
  S-Function/566 -> Bus Creator1/566  "enableWearF"
  S-Function/567 -> Bus Creator1/567  "nomBetaF"
  S-Function/568 -> Bus Creator1/568  "vWearR"
  S-Function/569 -> Bus Creator1/569  "nPowerWearR"
  S-Function/570 -> Bus Creator1/570  "nomTreadHeightR"
  S-Function/571 -> Bus Creator1/571  "alphaWFacR"
  S-Function/572 -> Bus Creator1/572  "kappaWFacR"
  S-Function/573 -> Bus Creator1/573  "camberWFacR"
  S-Function/574 -> Bus Creator1/574  "muxWEARR"
  S-Function/575 -> Bus Creator1/575  "ckappaWEARR"
  S-Function/576 -> Bus Creator1/576  "muyWEARR"
  S-Function/577 -> Bus Creator1/577  "cfalphaWEARR"
  S-Function/578 -> Bus Creator1/578  "enableWearR"
  S-Function/579 -> Bus Creator1/579  "nomBetaR"
  S-Function/580 -> Bus Creator1/580  "tyreTConTrackF"
  S-Function/581 -> Bus Creator1/581  "tyreTConTrackR"
  S-Function/582 -> Bus Creator1/582  "tyreTtrackF"
  S-Function/583 -> Bus Creator1/583  "tyreTtrackR"
  S-Function/584 -> Bus Creator1/584  "tyreHeatFluxFactorF"
  S-Function/585 -> Bus Creator1/585  "tyreHeatFluxFactorR"
  S-Function/586 -> Bus Creator1/586  "brakeInputMode"
  S-Function/587 -> Bus Creator1/587  "brakeSystemMode"
  S-Function/588 -> Bus Creator1/588  "brakeEnableTempF"
  S-Function/589 -> Bus Creator1/589  "brakeEnableTempR"
  S-Function/590 -> Bus Creator1/590  "brakeThresholdF"
  S-Function/591 -> Bus Creator1/591  "brakeThresholdR"
  S-Function/592 -> Bus Creator1/592  "brakeTMuFStart"
  S-Function/593 -> Bus Creator1/593  "brakeTMuRStart"
  S-Function/594 -> Bus Creator1/594  "clutchInertia"
  S-Function/595 -> Bus Creator1/595  "clutchEffR"
  S-Function/596 -> Bus Creator1/596  "clutchPeakNF"
  S-Function/597 -> Bus Creator1/597  "clutchMuStart"
  S-Function/598 -> Bus Creator1/598  "clutchMuEnd"
  S-Function/599 -> Bus Creator1/599  "engineDir"
  S-Function/600 -> Bus Creator1/600  "gearInertiaPrim"
  S-Function/601 -> Bus Creator1/601  "gearInertiaSec"
  S-Function/602 -> Bus Creator1/602  "diffInertiaAxleL"
  S-Function/603 -> Bus Creator1/603  "diffInertiaAxleR"
  S-Function/604 -> Bus Creator1/604  "diffEffTorqR0"
  S-Function/605 -> Bus Creator1/605  "diffEffTorqR1"
  S-Function/606 -> Bus Creator1/606  "diffEffTorqR2"
  S-Function/607 -> Bus Creator1/607  "diffPeakNF0"
  S-Function/608 -> Bus Creator1/608  "diffPeakNF1"
  S-Function/609 -> Bus Creator1/609  "diffPeakNF2"
  S-Function/610 -> Bus Creator1/610  "diffMuStart0"
  S-Function/611 -> Bus Creator1/611  "diffMuEnd0"
  S-Function/612 -> Bus Creator1/612  "aeroMode"
  S-Function/613 -> Bus Creator1/613  "aeroPxCOPUpright"
  S-Function/614 -> Bus Creator1/614  "aeroPyCOPUpright"
  S-Function/615 -> Bus Creator1/615  "aeroPzCOPUpright"
  S-Function/616 -> Bus Creator1/616  "driverMass"
  S-Function/617 -> Bus Creator1/617  "driverPosX"
  S-Function/618 -> Bus Creator1/618  "driverPosY"
  S-Function/619 -> Bus Creator1/619  "driverPosZ"
  S-Function/620 -> Bus Creator1/620  "driverInertiaX"
  S-Function/621 -> Bus Creator1/621  "driverInertiaY"
  S-Function/622 -> Bus Creator1/622  "driverInertiaZ"
  S-Function/623 -> Bus Creator1/623  "ballastMass"
  S-Function/624 -> Bus Creator1/624  "ballastPosX"
  S-Function/625 -> Bus Creator1/625  "ballastPosY"
  S-Function/626 -> Bus Creator1/626  "ballastPosZ"
  S-Function/627 -> Bus Creator1/627  "ballastInertiaX"
  S-Function/628 -> Bus Creator1/628  "ballastInertiaY"
  S-Function/629 -> Bus Creator1/629  "ballastInertiaZ"
  S-Function/630 -> Bus Creator1/630  "brakeTempMubFacF"
  S-Function/631 -> Bus Creator1/631  "brakeTempMubFacR"
  S-Function/632 -> Bus Creator1/632  "gearNeutralMode"
  S-Function/633 -> Bus Creator1/633  "gearReverseMode"
  S-Function/634 -> Bus Creator1/634  "steerMzFxFactor"
  S-Function/635 -> Bus Creator1/635  "steerMzFyFactor"
  Bus Creator1/1 -> imPar/1
  S-Function/636 -> Bus Creator1/636  "steerMzFzFactor"
  S-Function/637 -> Bus Creator1/637  "CSantiStallAcc"
  S-Function/638 -> Bus Creator1/638  "fuelTankPosx"
  S-Function/639 -> Bus Creator1/639  "fuelTankPosy"
  S-Function/640 -> Bus Creator1/640  "fuelTankPosz"
  S-Function/641 -> Bus Creator1/641  "brakeInputSig"
  S-Function/642 -> Bus Creator1/642  "engineAmbInflSel"
  S-Function/643 -> Bus Creator1/643  "engineAmbInflPress"
  S-Function/644 -> Bus Creator1/644  "engineAmbInflTemp"
  S-Function/645 -> Bus Creator1/645  "engineAmbInflHumid"
  S-Function/646 -> Bus Creator1/646  "CSpitLimEnableMap"
  S-Function/647 -> Bus Creator1/647  "suspLatWeightBalance"
  S-Function/648 -> Bus Creator1/648  "aeroDenSel"
  S-Function/649 -> Bus Creator1/649  "aeroAmbInflDenPress"
  S-Function/650 -> Bus Creator1/650  "aeroAmbInflDenTemp"
  S-Function/651 -> Bus Creator1/651  "fuelEnableMap"
  S-Function/652 -> Bus Creator1/652  "firstGearMode"
  S-Function/653 -> Bus Creator1/653  "shiftUpRPMLim"
  S-Function/654 -> Bus Creator1/654  "shiftDownRPMLim"
  S-Function/655 -> Bus Creator1/655  "scRpmLimDown"
  S-Function/656 -> Bus Creator1/656  "timeShiftMinUp"
  S-Function/657 -> Bus Creator1/657  "timeShiftMinDown"
  S-Function/658 -> Bus Creator1/658  "modeThrPulse"
  S-Function/659 -> Bus Creator1/659  "engineWOT"
  S-Function/660 -> Bus Creator1/660  "engineEnableStartAuto"
  S-Function/661 -> Bus Creator1/661  "engineStarterRatio"
  S-Function/662 -> Bus Creator1/662  "engineStarterRpmMax"
  S-Function/663 -> Bus Creator1/663  "engineStarterThr1"
  S-Function/664 -> Bus Creator1/664  "engineStarterThr2"
  S-Function/665 -> Bus Creator1/665  "engineStarterTD"
  S-Function/666 -> Bus Creator1/666  "engineEnablePowerSWAuto"
  S-Function/667 -> Bus Creator1/667  "clutchCalOff"
  S-Function/668 -> Bus Creator1/668  "clutchCalGain"
  S-Function/669 -> Bus Creator1/669  "roadInfo"
  S-Function/670 -> Bus Creator1/670  "suspEnableCenBumpCrvF"
  S-Function/671 -> Bus Creator1/671  "suspEnableCenBumpCrvR"
  S-Function/672 -> Bus Creator1/672  "suspEnableBumpCrvF"
  S-Function/673 -> Bus Creator1/673  "suspEnableBumpCrvR"
  S-Function/674 -> Bus Creator1/674  "suspNegCenBumpF"
  S-Function/675 -> Bus Creator1/675  "suspNegCenBumpR"
  S-Function/676 -> Bus Creator1/676  "suspNegBumpF"
  S-Function/677 -> Bus Creator1/677  "suspNegBumpR"
  S-Function/678 -> Bus Creator1/678  "suspRockerInertiaIxx0"
  S-Function/679 -> Bus Creator1/679  "suspRockerInertiaIxy0"
  S-Function/680 -> Bus Creator1/680  "suspRockerInertiaIxz0"
  S-Function/681 -> Bus Creator1/681  "suspRockerInertiaIyy0"
  S-Function/682 -> Bus Creator1/682  "suspRockerInertiaIyz0"
  S-Function/683 -> Bus Creator1/683  "suspRockerInertiaIzz0"
  S-Function/684 -> Bus Creator1/684  "suspRockerInertiaIxx1"
  S-Function/685 -> Bus Creator1/685  "suspRockerInertiaIxy1"
  S-Function/686 -> Bus Creator1/686  "suspRockerInertiaIxz1"
  S-Function/687 -> Bus Creator1/687  "suspRockerInertiaIyy1"
  S-Function/688 -> Bus Creator1/688  "suspRockerInertiaIyz1"
  S-Function/689 -> Bus Creator1/689  "suspRockerInertiaIzz1"
  S-Function/690 -> Bus Creator1/690  "suspRockerInertiaIxx2"
  S-Function/691 -> Bus Creator1/691  "suspRockerInertiaIxy2"
  S-Function/692 -> Bus Creator1/692  "suspRockerInertiaIxz2"
  S-Function/693 -> Bus Creator1/693  "suspRockerInertiaIyy2"
  S-Function/694 -> Bus Creator1/694  "suspRockerInertiaIyz2"
  S-Function/695 -> Bus Creator1/695  "suspRockerInertiaIzz2"
  S-Function/696 -> Bus Creator1/696  "suspRockerInertiaIxx3"
  S-Function/697 -> Bus Creator1/697  "suspRockerInertiaIxy3"
  S-Function/698 -> Bus Creator1/698  "suspRockerInertiaIxz3"
  S-Function/699 -> Bus Creator1/699  "suspRockerInertiaIyy3"
  S-Function/700 -> Bus Creator1/700  "suspRockerInertiaIyz3"
  S-Function/701 -> Bus Creator1/701  "suspRockerInertiaIzz3"
  S-Function/702 -> Bus Creator1/702  "suspUprightInertiaIxx0"
  S-Function/703 -> Bus Creator1/703  "suspUprightInertiaIxy0"
  S-Function/704 -> Bus Creator1/704  "suspUprightInertiaIxz0"
  S-Function/705 -> Bus Creator1/705  "suspUprightInertiaIyy0"
  S-Function/706 -> Bus Creator1/706  "suspUprightInertiaIyz0"
  S-Function/707 -> Bus Creator1/707  "suspUprightInertiaIzz0"
  S-Function/708 -> Bus Creator1/708  "suspUprightInertiaIxx1"
  S-Function/709 -> Bus Creator1/709  "suspUprightInertiaIxy1"
  S-Function/710 -> Bus Creator1/710  "suspUprightInertiaIxz1"
  S-Function/711 -> Bus Creator1/711  "suspUprightInertiaIyy1"
  S-Function/712 -> Bus Creator1/712  "suspUprightInertiaIyz1"
  S-Function/713 -> Bus Creator1/713  "suspUprightInertiaIzz1"
  S-Function/714 -> Bus Creator1/714  "suspUprightInertiaIxx2"
  S-Function/715 -> Bus Creator1/715  "suspUprightInertiaIxy2"
  S-Function/716 -> Bus Creator1/716  "suspUprightInertiaIxz2"
  S-Function/717 -> Bus Creator1/717  "suspUprightInertiaIyy2"
  S-Function/718 -> Bus Creator1/718  "suspUprightInertiaIyz2"
  S-Function/719 -> Bus Creator1/719  "suspUprightInertiaIzz2"
  S-Function/720 -> Bus Creator1/720  "suspUprightInertiaIxx3"
  S-Function/721 -> Bus Creator1/721  "suspUprightInertiaIxy3"
  S-Function/722 -> Bus Creator1/722  "suspUprightInertiaIxz3"
  S-Function/723 -> Bus Creator1/723  "suspUprightInertiaIyy3"
  S-Function/724 -> Bus Creator1/724  "suspUprightInertiaIyz3"
  S-Function/725 -> Bus Creator1/725  "suspUprightInertiaIzz3"
  S-Function/726 -> Bus Creator1/726  "suspRimInertiaIxx0"
  S-Function/727 -> Bus Creator1/727  "suspRimInertiaIxy0"
  S-Function/728 -> Bus Creator1/728  "suspRimInertiaIxz0"
  S-Function/729 -> Bus Creator1/729  "suspRimInertiaIyy0"
  S-Function/730 -> Bus Creator1/730  "suspRimInertiaIyz0"
  S-Function/731 -> Bus Creator1/731  "suspRimInertiaIzz0"
  S-Function/732 -> Bus Creator1/732  "suspRimInertiaIxx1"
  S-Function/733 -> Bus Creator1/733  "suspRimInertiaIxy1"
  S-Function/734 -> Bus Creator1/734  "suspRimInertiaIxz1"
  S-Function/735 -> Bus Creator1/735  "suspRimInertiaIyy1"
  S-Function/736 -> Bus Creator1/736  "suspRimInertiaIyz1"
  S-Function/737 -> Bus Creator1/737  "suspRimInertiaIzz1"
  S-Function/738 -> Bus Creator1/738  "suspRimInertiaIxx2"
  S-Function/739 -> Bus Creator1/739  "suspRimInertiaIxy2"
  S-Function/740 -> Bus Creator1/740  "suspRimInertiaIxz2"
  S-Function/741 -> Bus Creator1/741  "suspRimInertiaIyy2"
  S-Function/742 -> Bus Creator1/742  "suspRimInertiaIyz2"
  S-Function/743 -> Bus Creator1/743  "suspRimInertiaIzz2"
  S-Function/744 -> Bus Creator1/744  "suspRimInertiaIxx3"
  S-Function/745 -> Bus Creator1/745  "suspRimInertiaIxy3"
  S-Function/746 -> Bus Creator1/746  "suspRimInertiaIxz3"
  S-Function/747 -> Bus Creator1/747  "suspRimInertiaIyy3"
  S-Function/748 -> Bus Creator1/748  "suspRimInertiaIyz3"
  S-Function/749 -> Bus Creator1/749  "suspRimInertiaIzz3"
  S-Function/750 -> Bus Creator1/750  "suspRollInertiaFIxx"
  S-Function/751 -> Bus Creator1/751  "suspRollInertiaFIxy"
  S-Function/752 -> Bus Creator1/752  "suspRollInertiaFIxz"
  S-Function/753 -> Bus Creator1/753  "suspRollInertiaFIyy"
  S-Function/754 -> Bus Creator1/754  "suspRollInertiaFIyz"
  S-Function/755 -> Bus Creator1/755  "suspRollInertiaFIzz"
  S-Function/756 -> Bus Creator1/756  "suspRollInertiaRIxx"
  S-Function/757 -> Bus Creator1/757  "suspRollInertiaRIxy"
  S-Function/758 -> Bus Creator1/758  "suspRollInertiaRIxz"
  S-Function/759 -> Bus Creator1/759  "suspRollInertiaRIyy"
  S-Function/760 -> Bus Creator1/760  "suspRollInertiaRIyz"
  S-Function/761 -> Bus Creator1/761  "suspRollInertiaRIzz"
  S-Function/762 -> Bus Creator1/762  "tireInertiaIxx0"
  S-Function/763 -> Bus Creator1/763  "tireInertiaIxy0"
  S-Function/764 -> Bus Creator1/764  "tireInertiaIxz0"
  S-Function/765 -> Bus Creator1/765  "tireInertiaIyy0"
  S-Function/766 -> Bus Creator1/766  "tireInertiaIyz0"
  S-Function/767 -> Bus Creator1/767  "tireInertiaIzz0"
  S-Function/768 -> Bus Creator1/768  "tireInertiaIxx1"
  S-Function/769 -> Bus Creator1/769  "tireInertiaIxy1"
  S-Function/770 -> Bus Creator1/770  "tireInertiaIxz1"
  S-Function/771 -> Bus Creator1/771  "tireInertiaIyy1"
  S-Function/772 -> Bus Creator1/772  "tireInertiaIyz1"
  S-Function/773 -> Bus Creator1/773  "tireInertiaIzz1"
  S-Function/774 -> Bus Creator1/774  "tireInertiaIxx2"
  S-Function/775 -> Bus Creator1/775  "tireInertiaIxy2"
  S-Function/776 -> Bus Creator1/776  "tireInertiaIxz2"
  S-Function/777 -> Bus Creator1/777  "tireInertiaIyy2"
  S-Function/778 -> Bus Creator1/778  "tireInertiaIyz2"
  S-Function/779 -> Bus Creator1/779  "tireInertiaIzz2"
  S-Function/780 -> Bus Creator1/780  "tireInertiaIxx3"
  S-Function/781 -> Bus Creator1/781  "tireInertiaIxy3"
  S-Function/782 -> Bus Creator1/782  "tireInertiaIxz3"
  S-Function/783 -> Bus Creator1/783  "tireInertiaIyy3"
  S-Function/784 -> Bus Creator1/784  "tireInertiaIyz3"
  S-Function/785 -> Bus Creator1/785  "tireInertiaIzz3"
  S-Function/786 -> Bus Creator1/786  "bodyInertiaIxx"
  S-Function/787 -> Bus Creator1/787  "bodyInertiaIxy"
  S-Function/788 -> Bus Creator1/788  "bodyInertiaIxz"
  S-Function/789 -> Bus Creator1/789  "bodyInertiaIyy"
  S-Function/790 -> Bus Creator1/790  "bodyInertiaIyz"
  S-Function/791 -> Bus Creator1/791  "bodyInertiaIzz"
  S-Function/792 -> Bus Creator1/792  "engineInertiaIxx"
  S-Function/793 -> Bus Creator1/793  "engineInertiaIxy"
  S-Function/794 -> Bus Creator1/794  "engineInertiaIxz"
  S-Function/795 -> Bus Creator1/795  "engineInertiaIyy"
  S-Function/796 -> Bus Creator1/796  "engineInertiaIyz"
  S-Function/797 -> Bus Creator1/797  "engineInertiaIzz"
  S-Function/798 -> Bus Creator1/798  "driverInertiaIxx"
  S-Function/799 -> Bus Creator1/799  "driverInertiaIxy"
  S-Function/800 -> Bus Creator1/800  "driverInertiaIxz"
  S-Function/801 -> Bus Creator1/801  "driverInertiaIyy"
  S-Function/802 -> Bus Creator1/802  "driverInertiaIyz"
  S-Function/803 -> Bus Creator1/803  "driverInertiaIzz"
  S-Function/804 -> Bus Creator1/804  "ballastInertiaIxx"
  S-Function/805 -> Bus Creator1/805  "ballastInertiaIxy"
  S-Function/806 -> Bus Creator1/806  "ballastInertiaIxz"
  S-Function/807 -> Bus Creator1/807  "ballastInertiaIyy"
  S-Function/808 -> Bus Creator1/808  "ballastInertiaIyz"
  S-Function/809 -> Bus Creator1/809  "ballastInertiaIzz"
  S-Function/810 -> Bus Creator1/810  "steerrackInertiaIxx"
  S-Function/811 -> Bus Creator1/811  "steerrackInertiaIxy"
  S-Function/812 -> Bus Creator1/812  "steerrackInertiaIxz"
  S-Function/813 -> Bus Creator1/813  "steerrackInertiaIyy"
  S-Function/814 -> Bus Creator1/814  "steerrackInertiaIyz"
  S-Function/815 -> Bus Creator1/815  "steerrackInertiaIzz"
  S-Function/816 -> Bus Creator1/816  "engineCalThrOff"
  S-Function/817 -> Bus Creator1/817  "engineCalThrGain"
  S-Function/818 -> Bus Creator1/818  "CSpitLimSwMode"
  S-Function/819 -> Bus Creator1/819  "gearEffR"
  S-Function/820 -> Bus Creator1/820  "gearPeakNF"
  S-Function/821 -> Bus Creator1/821  "gearMuStart"
  S-Function/822 -> Bus Creator1/822  "gearMuEnd"
  S-Function/823 -> Bus Creator1/823  "tireEnableFilter"
  S-Function/824 -> Bus Creator1/824  "tireOmegaFilter"
  S-Function/825 -> Bus Creator1/825  "suspArbRockerPivotFx"
  S-Function/826 -> Bus Creator1/826  "suspArbRockerPivotFy"
  S-Function/827 -> Bus Creator1/827  "suspArbRockerPivotFz"
  S-Function/829 -> Bus Creator1/829  "suspArbRockerAxisFy"
  S-Function/828 -> Bus Creator1/828  "suspArbRockerAxisFx"
  S-Function/830 -> Bus Creator1/830  "suspArbRockerAxisFz"
  S-Function/831 -> Bus Creator1/831  "suspArbDroplinkRockerFx"
  S-Function/832 -> Bus Creator1/832  "suspArbDroplinkRockerFy"
  S-Function/833 -> Bus Creator1/833  "suspArbDroplinkRockerFz"
  S-Function/834 -> Bus Creator1/834  "suspArbDroplinkArbFx"
  S-Function/835 -> Bus Creator1/835  "suspArbDroplinkArbFy"
  S-Function/836 -> Bus Creator1/836  "suspArbDroplinkArbFz"
  S-Function/837 -> Bus Creator1/837  "suspArbRockerPivotRx"
  S-Function/838 -> Bus Creator1/838  "suspArbRockerPivotRy"
  S-Function/839 -> Bus Creator1/839  "suspArbRockerPivotRz"
  S-Function/840 -> Bus Creator1/840  "suspArbRockerAxisRx"
  S-Function/841 -> Bus Creator1/841  "suspArbRockerAxisRy"
  S-Function/842 -> Bus Creator1/842  "suspArbRockerAxisRz"
  S-Function/843 -> Bus Creator1/843  "suspArbDroplinkRockerRx"
  S-Function/844 -> Bus Creator1/844  "suspArbDroplinkRockerRy"
  S-Function/845 -> Bus Creator1/845  "suspArbDroplinkRockerRz"
  S-Function/846 -> Bus Creator1/846  "suspArbDroplinkArbRx"
  S-Function/847 -> Bus Creator1/847  "suspArbDroplinkArbRy"
  S-Function/848 -> Bus Creator1/848  "suspArbDroplinkArbRz"
  S-Function/849 -> Bus Creator1/849  "suspArbRockerMass0"
  S-Function/850 -> Bus Creator1/850  "suspArbRockerMass1"
  S-Function/851 -> Bus Creator1/851  "suspArbRockerMass2"
  S-Function/852 -> Bus Creator1/852  "suspArbRockerMass3"
  S-Function/853 -> Bus Creator1/853  "suspArbRockerInertiaIxx0"
  S-Function/854 -> Bus Creator1/854  "suspArbRockerInertiaIxy0"
  S-Function/855 -> Bus Creator1/855  "suspArbRockerInertiaIxz0"
  S-Function/856 -> Bus Creator1/856  "suspArbRockerInertiaIyy0"
  S-Function/857 -> Bus Creator1/857  "suspArbRockerInertiaIyz0"
  S-Function/858 -> Bus Creator1/858  "suspArbRockerInertiaIzz0"
  S-Function/859 -> Bus Creator1/859  "suspArbRockerInertiaIxx1"
  S-Function/863 -> Bus Creator1/863  "suspArbRockerInertiaIyz1"
  S-Function/862 -> Bus Creator1/862  "suspArbRockerInertiaIyy1"
  S-Function/861 -> Bus Creator1/861  "suspArbRockerInertiaIxz1"
  S-Function/860 -> Bus Creator1/860  "suspArbRockerInertiaIxy1"
  S-Function/866 -> Bus Creator1/866  "suspArbRockerInertiaIxy2"
  S-Function/865 -> Bus Creator1/865  "suspArbRockerInertiaIxx2"
  S-Function/864 -> Bus Creator1/864  "suspArbRockerInertiaIzz1"
  S-Function/869 -> Bus Creator1/869  "suspArbRockerInertiaIyz2"
  S-Function/868 -> Bus Creator1/868  "suspArbRockerInertiaIyy2"
  S-Function/867 -> Bus Creator1/867  "suspArbRockerInertiaIxz2"
  S-Function/895 -> Bus Creator1/895  "aeroSkidStiffFront"
  S-Function/894 -> Bus Creator1/894  "aeroSkidHeightRear"
  S-Function/893 -> Bus Creator1/893  "aeroSkidHeightFront"
  S-Function/892 -> Bus Creator1/892  "aeroDrsBrakeClose"
  S-Function/891 -> Bus Creator1/891  "aeroDrsThrottleClose"
  S-Function/890 -> Bus Creator1/890  "aeroDrsSteerOpen"
  S-Function/889 -> Bus Creator1/889  "aeroDrsAccyOpen"
  S-Function/870 -> Bus Creator1/870  "suspArbRockerInertiaIzz2"
  S-Function/871 -> Bus Creator1/871  "suspArbRockerInertiaIxx3"
  S-Function/872 -> Bus Creator1/872  "suspArbRockerInertiaIxy3"
  S-Function/873 -> Bus Creator1/873  "suspArbRockerInertiaIxz3"
  S-Function/874 -> Bus Creator1/874  "suspArbRockerInertiaIyy3"
  S-Function/875 -> Bus Creator1/875  "suspArbRockerInertiaIyz3"
  S-Function/876 -> Bus Creator1/876  "suspArbRockerInertiaIzz3"
  S-Function/877 -> Bus Creator1/877  "aeroBounceFrontOffset"
  S-Function/878 -> Bus Creator1/878  "aeroBounceRearOffset"
  S-Function/879 -> Bus Creator1/879  "aeroBounceThreshold1"
  S-Function/880 -> Bus Creator1/880  "aeroBounceThreshold2"
  S-Function/881 -> Bus Creator1/881  "aeroBounceSCZ1"
  S-Function/882 -> Bus Creator1/882  "aeroBounceSCZ2"
  S-Function/883 -> Bus Creator1/883  "aeroBounceDelay"
  S-Function/884 -> Bus Creator1/884  "aeroDrsCX"
  S-Function/885 -> Bus Creator1/885  "aeroDrsCZF"
  S-Function/886 -> Bus Creator1/886  "aeroDrsCZR"
  S-Function/887 -> Bus Creator1/887  "aeroDrsSpeedOpen"
  S-Function/888 -> Bus Creator1/888  "aeroDrsThrottleOpen"
  S-Function/896 -> Bus Creator1/896  "aeroSkidStiffRear"
  S-Function/897 -> Bus Creator1/897  "plate0x"
  S-Function/898 -> Bus Creator1/898  "plate0y"
  S-Function/899 -> Bus Creator1/899  "plate0z"
  S-Function/900 -> Bus Creator1/900  "plate1x"
  S-Function/901 -> Bus Creator1/901  "plate1y"
  S-Function/925 -> Bus Creator1/925  "suspStiffDeg3"
  S-Function/924 -> Bus Creator1/924  "suspStiffDeg2"
  S-Function/923 -> Bus Creator1/923  "suspStiffDeg1"
  S-Function/922 -> Bus Creator1/922  "suspStiffDeg0"
  S-Function/921 -> Bus Creator1/921  "plates"
  S-Function/920 -> Bus Creator1/920  "plate7z"
  S-Function/919 -> Bus Creator1/919  "plate7y"
  S-Function/918 -> Bus Creator1/918  "plate7x"
  S-Function/917 -> Bus Creator1/917  "plate6z"
  S-Function/916 -> Bus Creator1/916  "plate6y"
  S-Function/915 -> Bus Creator1/915  "plate6x"
  S-Function/914 -> Bus Creator1/914  "plate5z"
  S-Function/913 -> Bus Creator1/913  "plate5y"
  S-Function/912 -> Bus Creator1/912  "plate5x"
  S-Function/911 -> Bus Creator1/911  "plate4z"
  S-Function/910 -> Bus Creator1/910  "plate4y"
  S-Function/909 -> Bus Creator1/909  "plate4x"
  S-Function/908 -> Bus Creator1/908  "plate3z"
  S-Function/907 -> Bus Creator1/907  "plate3y"
  S-Function/906 -> Bus Creator1/906  "plate3x"
  S-Function/905 -> Bus Creator1/905  "plate2z"
  S-Function/904 -> Bus Creator1/904  "plate2y"
  S-Function/903 -> Bus Creator1/903  "plate2x"
  S-Function/902 -> Bus Creator1/902  "plate1z"
  S-Function/926 -> Bus Creator1/926  "suspThresholdDeg0"
